simulink model "Freescale_board"  (R2016a)
settings: Solver=FixedStepDiscrete  StartTime=0.0  StopTime=inf  RelTol=1e-3
libraries: frdmkl25zlib x10, frdmtfcshieldlib x5, simulink x3
settings Model: Creator=jkristof  LastModifiedBy=PBAOI
settings DataIOCC: LimitDataPoints=on  SaveFormat=Array
settings OptimizationCC: OptimizeModelRefInitCode=on  LifeSpan=1  MaxStackSize=64
settings DebuggingCC: SolverPrmCheckMsg=warning
settings HardwareCC: ProdBitPerPointer=32  ProdLargestAtomicInteger=Long  ProdLargestAtomicFloat=Double  ProdIntDivRoundTo=Undefined  ProdWordSize=32  ProdHWDeviceType=ARM Compatible->ARM Cortex
settings ModelReferenceCC: PropagateSignalLabelsOutOfModel=off
settings RTWCC: SystemTargetFile=ert.tlc  HardwareBoard=Freescale FRDM-KL25Z  TemplateMakefile=ert_default_tmf  Toolchain=GNU Tools for ARM Embedded Processors
settings CodeAppCC: IgnoreCustomStorageClasses=off
settings ERTTargetCC: ConvertIfToSwitch=off  SuppressUnreachableDefaultCases=off
settings ConfigComp: CovModelRefEnable=Off  CovSFcnEnable=off

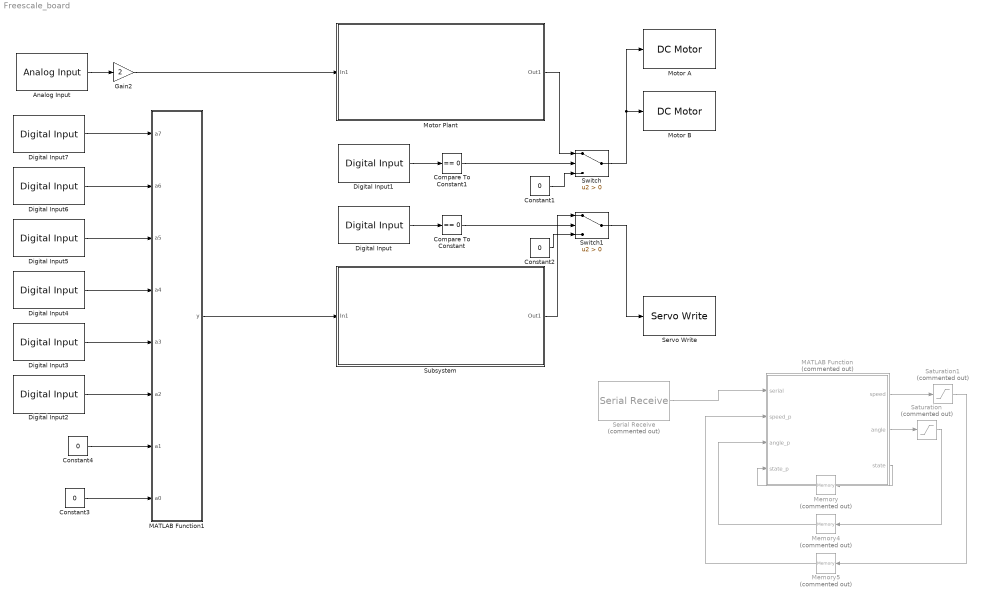
== system Freescale_board ==
  Analog Input : frdmkl25zlib/Analog Input  WhichPin=A1  SampleTime=0.0001
  Compare To Constant : simulink/Logic and Bit Operations/Compare To Constant  relop===  const=0  OutDataTypeStr=boolean
  Compare To Constant1 : simulink/Logic and Bit Operations/Compare To Constant  relop===  const=0  OutDataTypeStr=boolean
  Constant{1..4} (4 alike) : Constant  Value=0
  Digital Input : frdmkl25zlib/Digital Input  WhichPin=D0  SampleTime=0.0001
  Digital Input1 : frdmkl25zlib/Digital Input  WhichPin=D1  SampleTime=0.0001
  Digital Input2 : frdmkl25zlib/Digital Input  WhichPin=D2  SampleTime=0.0001
  Digital Input3 : frdmkl25zlib/Digital Input  WhichPin=D3  SampleTime=0.0001
  Digital Input4 : frdmkl25zlib/Digital Input  WhichPin=D4  SampleTime=0.0001
  Digital Input5 : frdmkl25zlib/Digital Input  WhichPin=D5  SampleTime=0.0001
  Digital Input6 : frdmkl25zlib/Digital Input  WhichPin=D6  SampleTime=0.0001
  Digital Input7 : frdmkl25zlib/Digital Input  WhichPin=D7  SampleTime=0.0001
  Gain2 : Gain  Gain=2
  MATLAB Function : MATLAB Function  Commented=on  TreatAsAtomicUnit=on
      settings: MinAlgLoopOccurrences=on
  MATLAB Function1 : MATLAB Function  TreatAsAtomicUnit=on
  Memory : Memory  Commented=on
  Memory4 : Memory  Commented=on
  Memory5 : Memory  Commented=on  X0=100
  "Motor A " : frdmtfcshieldlib/DC Motor  WhichMotor=A
  Motor B : frdmtfcshieldlib/DC Motor  WhichMotor=B
  Motor Plant : Subsystem
  Saturation : Saturate  Commented=on  UpperLimit=50  LowerLimit=0
  Saturation1 : Saturate  Commented=on  UpperLimit=200  LowerLimit=0
  Serial Receive : frdmkl25zlib/Serial Receive  Commented=on  uart=UART0  sampletime=0.00008681
  Servo Write : frdmtfcshieldlib/Servo Write  WhichServo=0  minAngle=-40  maxAngle=40
  Subsystem : Subsystem
  Switch : Switch  Criteria=u2 > Threshold
  Switch1 : Switch  Criteria=u2 > Threshold
  wires:
  Serial Receive/1 -> MATLAB Function/1(serial)
  Memory/1 -> MATLAB Function/4(state_p)
  Memory4/1 -> MATLAB Function/3(angle_p)
  Memory5/1 -> MATLAB Function/2(speed_p)
  MATLAB Function/3(state) -> Memory/1
  MATLAB Function/2(angle) -> Saturation/1
  Saturation/1 -> Memory4/1
  MATLAB Function/1(speed) -> Saturation1/1
  Saturation1/1 -> Memory5/1
  Digital Input7/1 -> MATLAB Function1/1(a7)
  Digital Input6/1 -> MATLAB Function1/2(a6)
  Digital Input5/1 -> MATLAB Function1/3(a5)
  Digital Input4/1 -> MATLAB Function1/4(a4)
  Digital Input3/1 -> MATLAB Function1/5(a3)
  Digital Input2/1 -> MATLAB Function1/6(a2)
  Gain2/1 -> Motor Plant/1(In1)
  Analog Input/1 -> Gain2/1
  MATLAB Function1/1(y) -> Subsystem/1(In1)
  Constant1/1 -> Switch/3
  Constant2/1 -> Switch1/3
  Motor Plant/1(Out1) -> Switch/1
  Switch/1 -> Motor B/1, "Motor A "/1
  Subsystem/1(Out1) -> Switch1/1
  Switch1/1 -> Servo Write/1
  Constant3/1 -> MATLAB Function1/8(a0)
  Digital Input/1 -> Compare To Constant/1
  Compare To Constant/1 -> Switch1/2
  Constant4/1 -> MATLAB Function1/7(a1)
  Digital Input1/1 -> Compare To Constant1/1
  Compare To Constant1/1 -> Switch/2

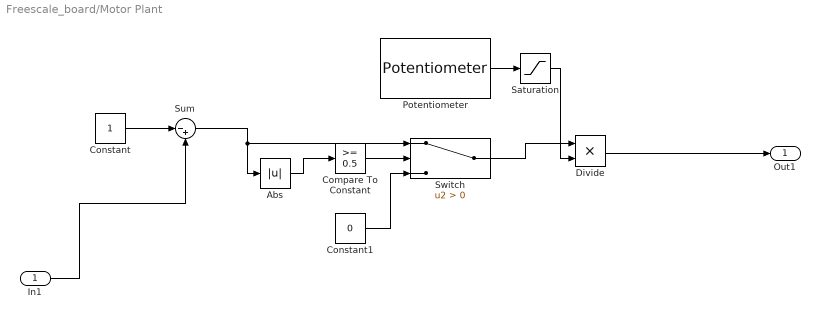
== system Freescale_board/Motor Plant ==
  In1 : Inport
  Abs : Abs
  Compare To Constant : simulink/Logic and Bit Operations/Compare To Constant  relop=>=  const=0.5  OutDataTypeStr=boolean
  Constant : Constant
  Constant1 : Constant  Value=0
  Divide : Product  Inputs=**
  Potentiometer : frdmtfcshieldlib/Potentiometer  WhichPot=A  SampleTime=0.0001
  Saturation : Saturate  UpperLimit=1  LowerLimit=0
  Sum : Sum  Inputs=|-+
  Switch : Switch  Criteria=u2 > Threshold
  Out1 : Outport
  wires:
  Constant/1 -> Sum/1
  In1/1 -> Sum/2
  Potentiometer/1 -> Saturation/1
  Sum/1 -> Switch/1, Abs/1
  Constant1/1 -> Switch/3
  Compare To Constant/1 -> Switch/2
  Abs/1 -> Compare To Constant/1
  Saturation/1 -> Divide/2
  Switch/1 -> Divide/1
  Divide/1 -> Out1/1

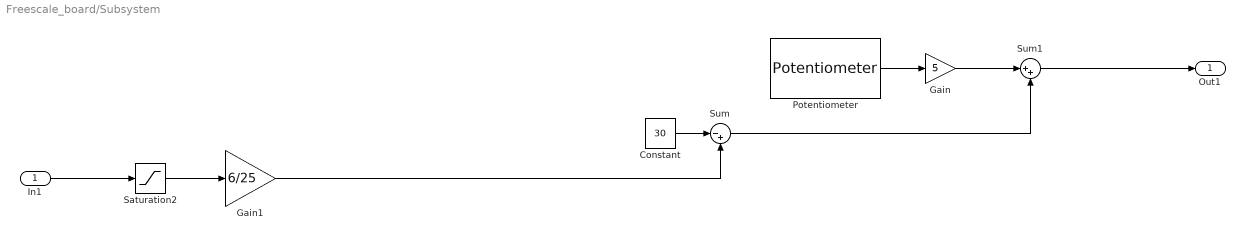
== system Freescale_board/Subsystem ==
  In1 : Inport
  Constant : Constant  Value=30
  Gain : Gain  Gain=5
  Gain1 : Gain  Gain=6/25
  Potentiometer : frdmtfcshieldlib/Potentiometer  WhichPot=B  SampleTime=0.0001
  Saturation2 : Saturate  UpperLimit=250  LowerLimit=0
  Sum : Sum  Inputs=|-+
  Sum1 : Sum  Inputs=|++
  Out1 : Outport
  wires:
  In1/1 -> Saturation2/1
  Saturation2/1 -> Gain1/1
  Gain1/1 -> Sum/2
  Sum/1 -> Sum1/2
  Potentiometer/1 -> Gain/1
  Constant/1 -> Sum/1
  Gain/1 -> Sum1/1
  Sum1/1 -> Out1/1

== matlab function Freescale_board/MATLAB Function1 ==
  data: a7 input; y output; a6 input; a5 input; a4 input; a3 input; a2 input; a1 input; a0 input
function  y = fcn(a7,a6,a5,a4,a3,a2,a1,a0)
%#codegen

y = (a7*2^7)+(a6*2^6)+(a5*2^5)+(a4*2^4)+(a3*2^3)+(a2*2^2)+(a1*2^1)+(a0*2^0);

== matlab function Freescale_board/MATLAB Function ==
  data: speed output; serial input; speed_p input; angle_p input; angle output; state_p input; state output
function [speed,angle,state]= fcn(serial,speed_p,angle_p,state_p)
%#codegen
state = state_p;
speed = speed_p;
angle = angle_p;
if(state ==1)
    speed = double(serial);
    state = 0;
elseif(state ==2)
    angle = double(serial);
    state = 0;
end
if(serial == 83 && state == 0)%'S'
    state = 1;
elseif(serial == 65 && state == 0)%'A'
    state = 2;

end
